simulink model "sum_collapse_bool_test"  (Simulink 7.2)
settings: Solver=VariableStepDiscrete  StartTime=0.0  StopTime=10.0  RelTol=1e-3
settings Model: Creator=arnaud  LastModifiedBy=arnaud
settings DataIOCC: SaveFormat=Structure

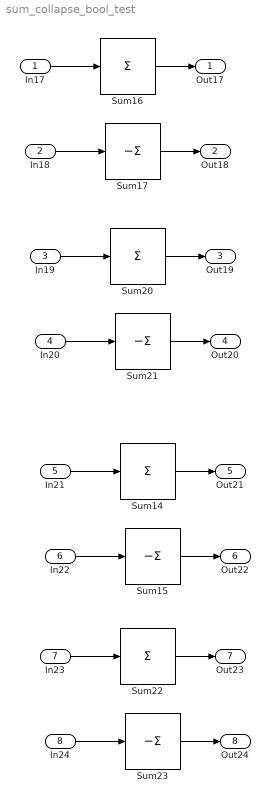
== system sum_collapse_bool_test ==
  In17 : Inport  DataType=boolean  OutDataType=sfix(16)  OutScaling=2^0  OutDataTypeStr=boolean
  In18 : Inport  Port=2  DataType=boolean  OutDataType=sfix(16)  OutScaling=2^0  OutDataTypeStr=boolean
  In19 : Inport  Port=3  PortDimensions=3  DataType=boolean  OutDataType=sfix(16)  OutScaling=2^0  OutDataTypeStr=boolean
  In20 : Inport  Port=4  PortDimensions=3  DataType=boolean  OutDataType=sfix(16)  OutScaling=2^0  OutDataTypeStr=boolean
  In21 : Inport  Port=5  PortDimensions=[2 3]  DataType=boolean  OutDataType=sfix(16)  OutScaling=2^0  OutDataTypeStr=boolean
  In22 : Inport  Port=6  PortDimensions=[2 3]  DataType=boolean  OutDataType=sfix(16)  OutScaling=2^0  OutDataTypeStr=boolean
  In23 : Inport  Port=7  PortDimensions=[2 3]  DataType=boolean  OutDataType=sfix(16)  OutScaling=2^0  OutDataTypeStr=boolean
  In24 : Inport  Port=8  PortDimensions=[2 3]  DataType=boolean  OutDataType=sfix(16)  OutScaling=2^0  OutDataTypeStr=boolean
  Sum14 : Sum  Inputs=+  CollapseMode=Specified dimension  OutDataType=sfix(16)  OutScaling=2^0
  Sum15 : Sum  Inputs=-  CollapseMode=Specified dimension  OutDataType=sfix(16)  OutScaling=2^0
  Sum16 : Sum  Inputs=+  CollapseMode=Specified dimension  OutDataType=sfix(16)  OutScaling=2^0
  Sum17 : Sum  Inputs=-  CollapseMode=Specified dimension  OutDataType=sfix(16)  OutScaling=2^0
  Sum20 : Sum  Inputs=+  CollapseMode=Specified dimension  OutDataType=sfix(16)  OutScaling=2^0
  Sum21 : Sum  Inputs=-  CollapseMode=Specified dimension  OutDataType=sfix(16)  OutScaling=2^0
  Sum22 : Sum  Inputs=+  CollapseMode=Specified dimension  CollapseDim=2  OutDataType=sfix(16)  OutScaling=2^0
  Sum23 : Sum  Inputs=-  CollapseMode=Specified dimension  CollapseDim=2  OutDataType=sfix(16)  OutScaling=2^0
  Out17 : Outport  OutDataType=sfix(16)  OutScaling=2^0
  Out18 : Outport  Port=2  OutDataType=sfix(16)  OutScaling=2^0
  Out19 : Outport  Port=3  OutDataType=sfix(16)  OutScaling=2^0
  Out20 : Outport  Port=4  OutDataType=sfix(16)  OutScaling=2^0
  Out21 : Outport  Port=5  OutDataType=sfix(16)  OutScaling=2^0
  Out22 : Outport  Port=6  OutDataType=sfix(16)  OutScaling=2^0
  Out23 : Outport  Port=7  OutDataType=sfix(16)  OutScaling=2^0
  Out24 : Outport  Port=8  OutDataType=sfix(16)  OutScaling=2^0
  wires:
  In17/1 -> Sum16/1
  Sum16/1 -> Out17/1
  In18/1 -> Sum17/1
  Sum17/1 -> Out18/1
  In19/1 -> Sum20/1
  Sum20/1 -> Out19/1
  In20/1 -> Sum21/1
  Sum21/1 -> Out20/1
  In21/1 -> Sum14/1
  Sum14/1 -> Out21/1
  In22/1 -> Sum15/1
  Sum15/1 -> Out22/1
  In23/1 -> Sum22/1
  Sum22/1 -> Out23/1
  In24/1 -> Sum23/1
  Sum23/1 -> Out24/1
